simulink model "Simulator_Case_9"  (R2024a)
settings: Solver=VariableStepAuto  StartTime=0.0  StopTime=1400  RelTol=1e-3
values from neighbouring files (symbols this model uses):
  Declination_Sigean = 2.116*(pi/180)    (= 0.0369311669722)    [Parametrization_Simulation_Case_9.m]
  Position_Initial_X = Waypoints_X(1)    [Parametrization_Simulation_Case_9.m]
  Position_Initial_Y = Waypoints_Y(1)    [Parametrization_Simulation_Case_9.m]
  Time_Period_Sampling = 0.1    [Parametrization_Simulation_Case_9.m]
  Velocity_Norm_Ship_Initial = 6/3.6    (= 1.66666666667)    [Parametrization_Simulation_Case_9.m]
undefined symbols (not defined in the file or in its folder): Damping_Coefficient, Damping_Factor_Waves, Density_Water_Salted, Draft_Depth, Drag_Coefficient, Gain_Filter, Inertia_Moment, Length_Ship, Longeron_Area, Mass_Ship, Pulsation_Natural, Pulsation_Wave, Rudder_Angle_Maximal, Rudder_Angle_Minimal, Rudder_Rate_Maximal, Rudder_Rate_Minimal, Static_Gain_Nomoto, Time_Constant_Total, Waypoints
libraries: cstblocks x2, simulink_extras x1
(part 1 of 2)
settings Model: Creator=gerar  LastModifiedBy=gerar
settings DebuggingCC: UnderSpecifiedDimensionMsg=warning

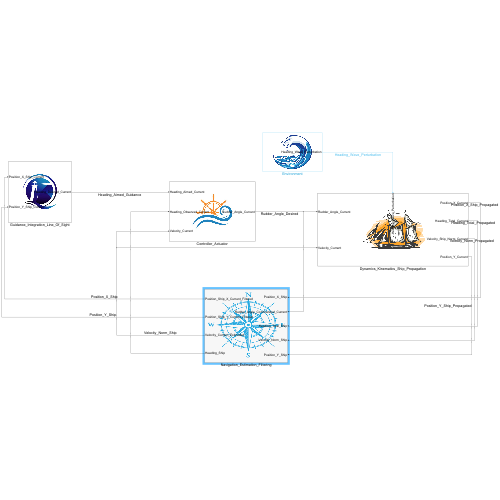
[thumbnail: Simulink's stored preview of the top-level diagram]
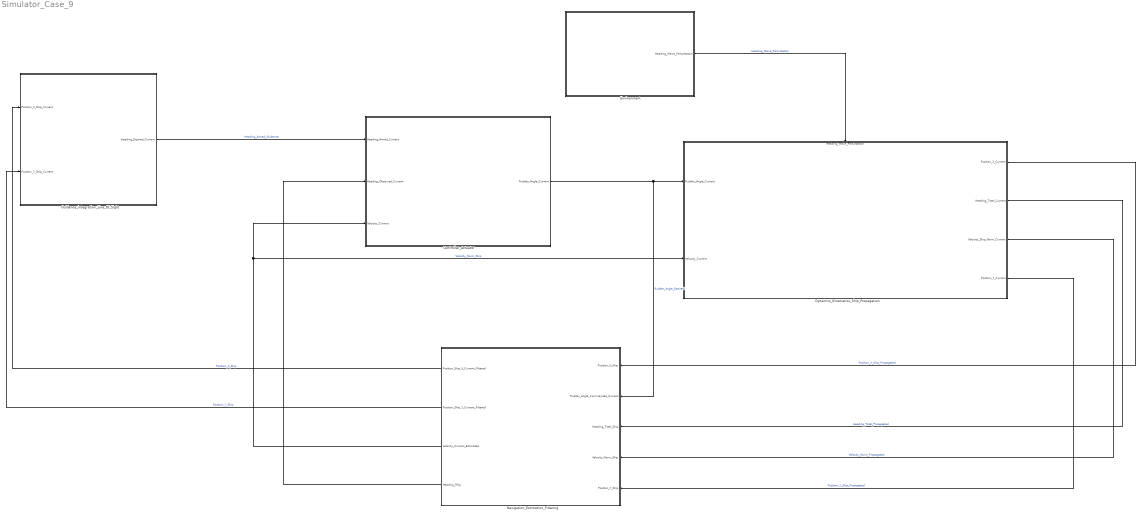
== system Simulator_Case_9 ==
  Controller_Actuator : Subsystem
      mask Display: image('Rudder3.jpg');
  Dynamics_Kinematics_Ship_Propagation : Subsystem
      settings: PortSchema="{\"entries\":[{\"content\":{\"sides\":[{\"content\":{\"connectorIds\":[\"In1\",\"In2\"]},\"type\":\"ConnectorPlacement.EquallySpacedRectSide\",\"uuid\":\"15ab685c-7974-4319-9f6c-957ada7f76c2\"},{\"content\":{\"connectorIds\":[\"Out1\",\"Out2\",\"Out3\",\"Out4\"],\"side\":\"RIGHT\"},\"type\":\"ConnectorPlacement.EquallySpacedRectSide\",\"uuid\":\"012aae79-88c5-42c2-86b9-e231f4da87b9\"},{\"content\":{\"connectorIds\":[\"In3\"],\"side\":\"TOP\"},\"type\":\"ConnectorPlacement.EquallySpacedRectSide\",\"uuid\":\"7672cff3-9f29-4819-a889-c5ff0e6add92\"}]},\"type\":\"ConnectorPlacement.EquallySpacedConnector\",\"uuid\":\"ccb47c3f-4c98-48cb-bcca-80a3d04d13a2\"}],\"packageUris\":[\"http://schema.mathworks.com/mf0/Connector/R2020b\"],\"version\":\"1.0\"}"
      mask Display: image('ship2.png');
  Environment : Subsystem
      mask Display: image('Wave2.png');
  Guidance_Integration_Line_Of_Sight : Subsystem
      mask Display: image('phare4.jpg');
  Navigation_Estimation_Filtering : Subsystem
      mask Display: image('compass4.png');
  wires:
  Navigation_Estimation_Filtering/1(Position_Ship_X_Current_Filtered) -> Guidance_Integration_Line_Of_Sight/1(Position_X_Ship_Current)  "Position_X_Ship"
  Navigation_Estimation_Filtering/2(Position_Ship_Y_Current_Filtered) -> Guidance_Integration_Line_Of_Sight/2(Position_Y_Ship_Current)  "Position_Y_Ship"
  Guidance_Integration_Line_Of_Sight/1(Heading_Desired_Current) -> Controller_Actuator/1(Heading_Aimed_Current)  "Heading_Aimed_Guidance"
  Navigation_Estimation_Filtering/3(Velocity_Current_Estimated) -> Dynamics_Kinematics_Ship_Propagation/2(Velocity_Current), Controller_Actuator/3(Velocity_Current)  "Velocity_Norm_Ship"
  Controller_Actuator/1(Rudder_Angle_Current) -> Navigation_Estimation_Filtering/2(Rudder_Angle_Commanded_Current), Dynamics_Kinematics_Ship_Propagation/1(Rudder_Angle_Current)  "Rudder_Angle_Desired"
  Environment/1(Heading_Wave_Perturbation) -> Dynamics_Kinematics_Ship_Propagation/3(Heading_Wave_Perturbation)  "Heading_Wave_Perturbation"
  Dynamics_Kinematics_Ship_Propagation/1(Position_X_Current) -> Navigation_Estimation_Filtering/1(Position_X_Ship)  "Position_X_Ship_Propagated"
  Dynamics_Kinematics_Ship_Propagation/2(Heading_Total_Current) -> Navigation_Estimation_Filtering/3(Heading_Total_Ship)  "Heading_Total_Propagated"
  Dynamics_Kinematics_Ship_Propagation/3(Velocity_Ship_Norm_Current) -> Navigation_Estimation_Filtering/4(Velocity_Norm_Ship)  "Velocity_Norm_Propagated"
  Dynamics_Kinematics_Ship_Propagation/4(Position_Y_Current) -> Navigation_Estimation_Filtering/5(Position_Y_Ship)  "Position_Y_Ship_Propagated"
  Navigation_Estimation_Filtering/4(Heading_Ship) -> Controller_Actuator/2(Heading_Observed_Current)

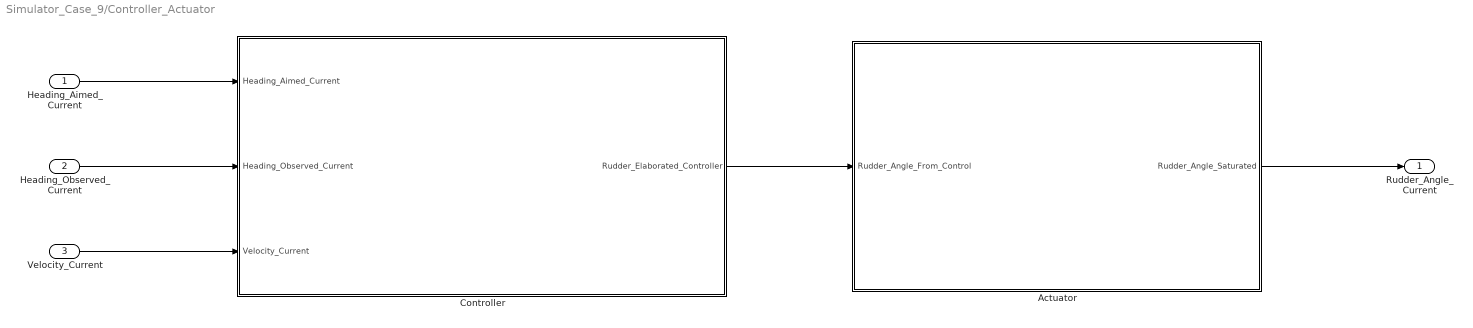
== system Simulator_Case_9/Controller_Actuator ==
  Heading_Aimed_Current : Inport
  Heading_Observed_Current : Inport  Port=2
  Velocity_Current : Inport  Port=3
  Actuator : Subsystem
  Controller : Subsystem
  Rudder_Angle_Current : Outport
  wires:
  Heading_Aimed_Current/1 -> Controller/1(Heading_Aimed_Current)
  Heading_Observed_Current/1 -> Controller/2(Heading_Observed_Current)
  Velocity_Current/1 -> Controller/3(Velocity_Current)
  Controller/1(Rudder_Elaborated_Controller) -> Actuator/1(Rudder_Angle_From_Control)
  Actuator/1(Rudder_Angle_Saturated) -> Rudder_Angle_Current/1

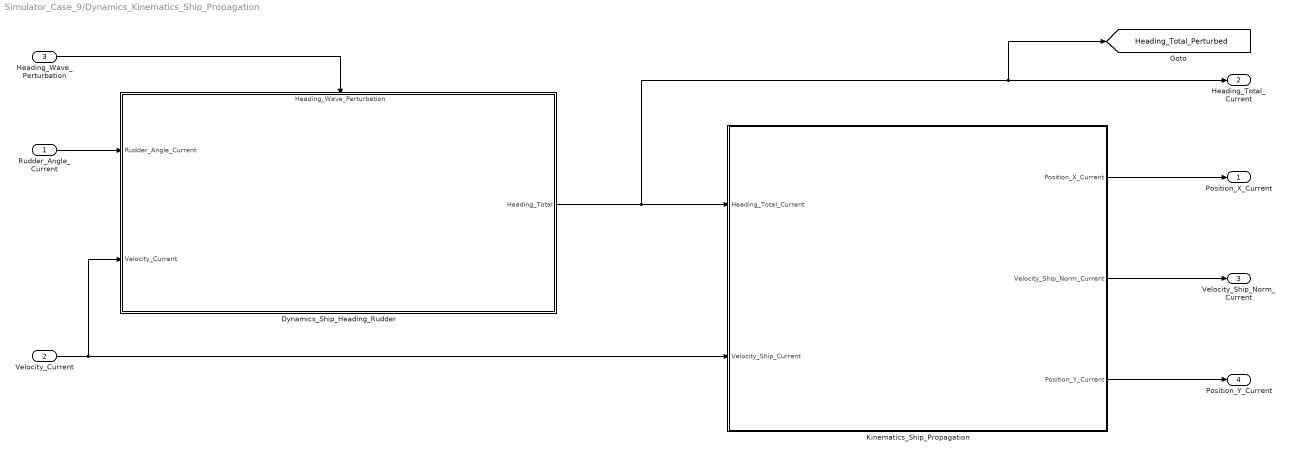
== system Simulator_Case_9/Dynamics_Kinematics_Ship_Propagation ==
  Rudder_Angle_Current : Inport
  Velocity_Current : Inport  Port=2
  Heading_Wave_Perturbation : Inport  Port=3
  Dynamics_Ship_Heading_Rudder : Subsystem
      settings: PortSchema="{\"entries\":[{\"content\":{\"sides\":[{\"content\":{\"connectorIds\":[\"In1\",\"In2\"]},\"type\":\"ConnectorPlacement.EquallySpacedRectSide\",\"uuid\":\"5eab7870-9471-4536-8507-22041873c494\"},{\"content\":{\"connectorIds\":[\"Out1\"],\"side\":\"RIGHT\"},\"type\":\"ConnectorPlacement.EquallySpacedRectSide\",\"uuid\":\"f266833a-c986-4c85-b5bf-5f6330a2f0dc\"},{\"content\":{\"connectorIds\":[\"In3\"],\"side\":\"TOP\"},\"type\":\"ConnectorPlacement.EquallySpacedRectSide\",\"uuid\":\"9dc2f366-9cc9-4ae6-8111-85e400a47094\"}]},\"type\":\"ConnectorPlacement.EquallySpacedConnector\",\"uuid\":\"570359d0-6206-4da5-90c2-7e8bebb6ea91\"}],\"packageUris\":[\"http://schema.mathworks.com/mf0/Connector/R2020b\"],\"version\":\"1.0\"}"
  Kinematics_Ship_Propagation : Subsystem
  Position_X_Current : Outport
  Heading_Total_Current : Outport  Port=2
  Velocity_Ship_Norm_Current : Outport  Port=3
  Position_Y_Current : Outport  Port=4
  tag scope: Heading_Total_Perturbed=global
  wires:
  Dynamics_Ship_Heading_Rudder/1(Heading_Total) -> [Heading_Total_Perturbed], Heading_Total_Current/1, Kinematics_Ship_Propagation/1(Heading_Total_Current)
  Kinematics_Ship_Propagation/1(Position_X_Current) -> Position_X_Current/1
  Velocity_Current/1 -> Kinematics_Ship_Propagation/2(Velocity_Ship_Current), Dynamics_Ship_Heading_Rudder/2(Velocity_Current)
  Rudder_Angle_Current/1 -> Dynamics_Ship_Heading_Rudder/1(Rudder_Angle_Current)
  Heading_Wave_Perturbation/1 -> Dynamics_Ship_Heading_Rudder/3(Heading_Wave_Perturbation)
  Kinematics_Ship_Propagation/3(Position_Y_Current) -> Position_Y_Current/1
  Kinematics_Ship_Propagation/2(Velocity_Ship_Norm_Current) -> Velocity_Ship_Norm_Current/1

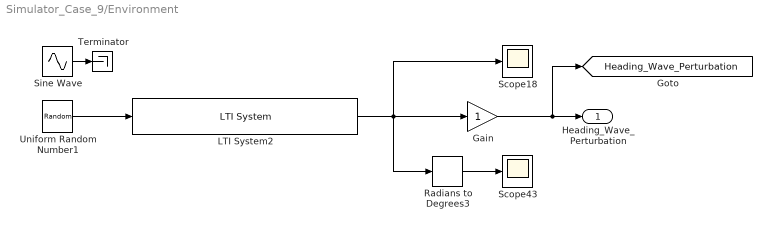
== system Simulator_Case_9/Environment ==
  Gain : Gain
  LTI System2 : cstblocks/LTI System  sys=Wave_Transfer_Function  IC=[]  PadeOrder=0
  Radians to Degrees3 : simulink_extras/Transformations/Radians to Degrees
  Scope18 : Scope
  Scope43 : Scope
  Sine Wave : Sin  Amplitude=6*(pi/180)  Frequency=1.2  SampleTime=0
  Terminator : Terminator
  Uniform Random Number1 : UniformRandomNumber  Minimum=-17*(pi/180)  Maximum=17*(pi/180)  SampleTime=Time_Period_Sampling
  Heading_Wave_Perturbation : Outport
  tag scope: Heading_Wave_Perturbation=global
  wires:
  LTI System2/1 -> Gain/1, Radians to Degrees3/1, Scope18/1
  Radians to Degrees3/1 -> Scope43/1
  Gain/1 -> [Heading_Wave_Perturbation], Heading_Wave_Perturbation/1
  Uniform Random Number1/1 -> LTI System2/1
  Sine Wave/1 -> Terminator/1

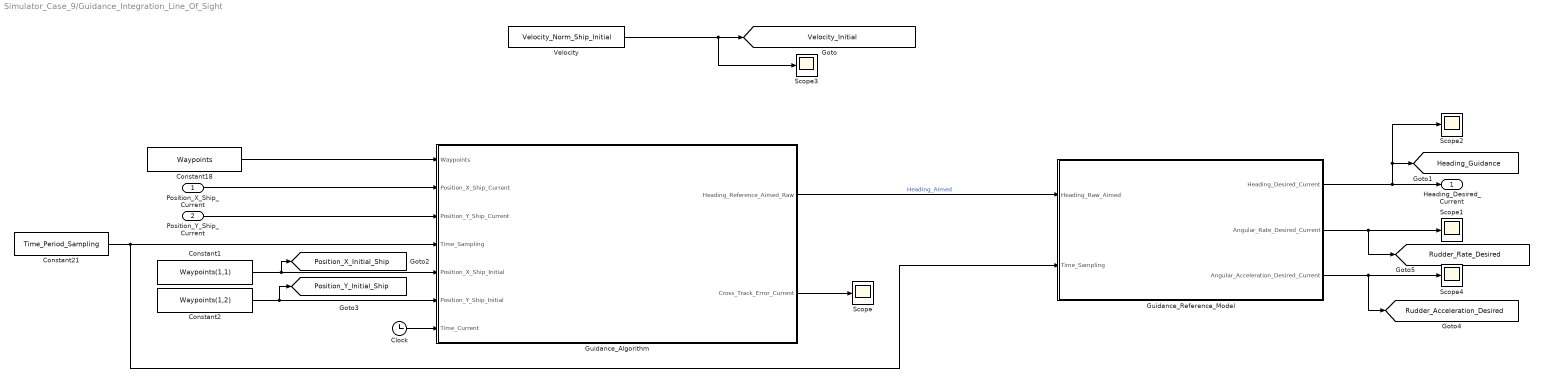
== system Simulator_Case_9/Guidance_Integration_Line_Of_Sight ==
  Position_X_Ship_Current : Inport
  Position_Y_Ship_Current : Inport  Port=2
  Clock : Clock
  Constant1 : Constant  Value=Waypoints(1,1)
  Constant18 : Constant  Value=Waypoints
  Constant2 : Constant  Value=Waypoints(1,2)
  Constant21 : Constant  Value=Time_Period_Sampling
  Guidance_Algorithm : MATLAB Function  TreatAsAtomicUnit=on  SystemSampleTime=Time_Period_Sampling
  Guidance_Reference_Model : MATLAB Function  TreatAsAtomicUnit=on  SystemSampleTime=Time_Period_Sampling
  Scope{,1..4} (5 alike) : Scope
  Velocity : Constant  Value=Velocity_Norm_Ship_Initial
  Heading_Desired_Current : Outport
  tag scope: Heading_Guidance=global, Position_X_Initial_Ship=global, Position_Y_Initial_Ship=global, Rudder_Acceleration_Desired=global, Rudder_Rate_Desired=global, Velocity_Initial=global
  wires:
  Guidance_Algorithm/2(Cross_Track_Error_Current) -> Scope/1
  Constant21/1 -> Guidance_Algorithm/4(Time_Sampling), Guidance_Reference_Model/2(Time_Sampling)
  Guidance_Reference_Model/2(Angular_Rate_Desired_Current) -> [Rudder_Rate_Desired], Scope1/1
  Constant18/1 -> Guidance_Algorithm/1(Waypoints)
  Guidance_Algorithm/1(Heading_Reference_Aimed_Raw) -> Guidance_Reference_Model/1(Heading_Raw_Aimed)  "Heading_Aimed"
  Guidance_Reference_Model/1(Heading_Desired_Current) -> Heading_Desired_Current/1, Scope2/1, [Heading_Guidance]
  Position_Y_Ship_Current/1 -> Guidance_Algorithm/3(Position_Y_Ship_Current)
  Position_X_Ship_Current/1 -> Guidance_Algorithm/2(Position_X_Ship_Current)
  Constant1/1 -> [Position_X_Initial_Ship], Guidance_Algorithm/5(Position_X_Ship_Initial)
  Constant2/1 -> [Position_Y_Initial_Ship], Guidance_Algorithm/6(Position_Y_Ship_Initial)
  Clock/1 -> Guidance_Algorithm/7(Time_Current)
  Velocity/1 -> Scope3/1, [Velocity_Initial]
  Guidance_Reference_Model/3(Angular_Acceleration_Desired_Current) -> [Rudder_Acceleration_Desired], Scope4/1

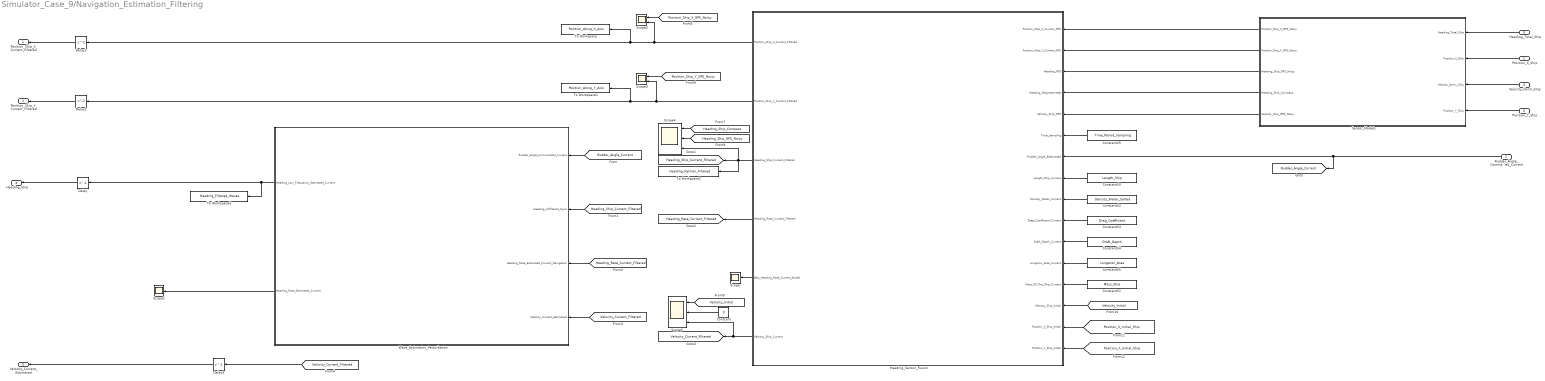
== system Simulator_Case_9/Navigation_Estimation_Filtering ==
  Position_X_Ship : Inport
  Rudder_Angle_Commanded_Current : Inport  Port=2
  Heading_Total_Ship : Inport  Port=3
  Velocity_Norm_Ship : Inport  Port=4
  Position_Y_Ship : Inport  Port=5
  Constant : Constant  Value=0
  Constant25 : Constant  Value=Time_Period_Sampling
  Constant50 : Constant  Value=Length_Ship
  Constant51 : Constant  Value=Mass_Ship
  Constant52 : Constant  Value=Density_Water_Salted
  Constant53 : Constant  Value=Drag_Coefficient
  Constant54 : Constant  Value=Draft_Depth
  Constant55 : Constant  Value=Longeron_Area
  Delay{,1..3} (4 alike) : Delay  DelayLength=1  InputProcessing=Columns as channels (frame based)  SampleTime=Time_Period_Sampling
  Heading_Sensor_Fusion : MATLAB Function  TreatAsAtomicUnit=on  SystemSampleTime=Time_Period_Sampling
  Scope : Scope
  Scope1 : Scope
  Scope2 : Scope  NumInputPorts=2
  Scope3 : Scope  NumInputPorts=2
  Scope4 : Scope  NumInputPorts=3
  Scope5 : Scope  NumInputPorts=3
  Sensor_Models : Subsystem
  To Workspace : ToWorkspace  VariableName=Position_Along_X_Axis  SaveFormat=Timeseries  SampleTime=-1
  To Workspace1 : ToWorkspace  VariableName=Position_Along_Y_Axis  SaveFormat=Timeseries  SampleTime=-1
  To Workspace2 : ToWorkspace  VariableName=Heading_Kalman_Filtered  SaveFormat=Timeseries  SampleTime=-1
  To Workspace3 : ToWorkspace  VariableName=Heading_Filtered_Waves  SaveFormat=Timeseries  SampleTime=-1
  Wave_Estimation_Perturbation : Subsystem
  Position_Ship_X_Current_Filtered : Outport
  Position_Ship_Y_Current_Filtered : Outport  Port=2
  Velocity_Current_Estimated : Outport  Port=3
  Heading_Ship : Outport  Port=4
  tag scope: Heading_Rate_Current_Filtered=global, Heading_Ship_Current_Filtered=global, Rudder_Angle_Current=global, Velocity_Current_Filtered=global
  wires:
  Heading_Sensor_Fusion/5(Bias_Heading_Rate_Current_Model) -> Scope/1
  Heading_Total_Ship/1 -> Sensor_Models/1(Heading_Total_Ship)
  Constant25/1 -> Heading_Sensor_Fusion/6(Time_Sampling)
  Constant55/1 -> Heading_Sensor_Fusion/12(Longeron_Area_Current)
  Sensor_Models/4(Heading_Ship_Compass) -> Heading_Sensor_Fusion/4(Heading_Magnetometer)
  Constant51/1 -> Heading_Sensor_Fusion/13(Mass_Of_The_Ship_Current)
  Sensor_Models/1(Position_Ship_X_GPS_Noisy) -> Heading_Sensor_Fusion/1(Position_Ship_X_Current_GPS)
  Sensor_Models/2(Position_Ship_Y_GPS_Noisy) -> Heading_Sensor_Fusion/2(Position_Ship_Y_Current_GPS)
  Velocity_Norm_Ship/1 -> Sensor_Models/3(Velocity_Norm_Ship)
  Sensor_Models/3(Heading_Ship_GPS_Noisy) -> Heading_Sensor_Fusion/3(Heading_GPS)
  Sensor_Models/5(Velocity_Ship_GPS_Noisy) -> Heading_Sensor_Fusion/5(Velocity_Ship_GPS)
  Constant54/1 -> Heading_Sensor_Fusion/11(Draft_Depth_Current)
  Constant50/1 -> Heading_Sensor_Fusion/8(Length_Ship_Current)
  Position_X_Ship/1 -> Sensor_Models/2(Position_X_Ship)
  Constant52/1 -> Heading_Sensor_Fusion/9(Density_Water_Current)
  Constant53/1 -> Heading_Sensor_Fusion/10(Drag_Coefficient_Current)
  Wave_Estimation_Perturbation/2(Heading_Rate_Estimated_Current) -> Scope1/1
  Wave_Estimation_Perturbation/1(Heading_Low_Frequency_Estimated_Current) -> To Workspace3/1, Delay/1
  Heading_Sensor_Fusion/2(Position_Ship_Y_Current_Filtered) -> Scope3/2, To Workspace1/1, Delay2/1
  Heading_Sensor_Fusion/1(Position_Ship_X_Current_Filtered) -> Scope2/2, To Workspace/1, Delay1/1
  Rudder_Angle_Commanded_Current/1 -> [Rudder_Angle_Current], Heading_Sensor_Fusion/7(Rudder_Angle_Elaborated)
  Position_Y_Ship/1 -> Sensor_Models/4(Position_Y_Ship)
  [Rudder_Angle_Current] -> Wave_Estimation_Perturbation/1(Rudder_Angle_Commanded_Current)
  Heading_Sensor_Fusion/3(Heading_Ship_Current_Filtered) -> To Workspace2/1, Scope4/3, [Heading_Ship_Current_Filtered]
  [Heading_Ship_Current_Filtered] -> Wave_Estimation_Perturbation/2(Heading_Unfiltered_Input)
  Heading_Sensor_Fusion/4(Heading_Rate_Current_Filtered) -> [Heading_Rate_Current_Filtered]
  [Heading_Rate_Current_Filtered] -> Wave_Estimation_Perturbation/3(Heading_Rate_Estimated_Current_Navigation)
  Heading_Sensor_Fusion/6(Velocity_Ship_Current) -> Scope5/3, [Velocity_Current_Filtered]
  [Velocity_Current_Filtered] -> Wave_Estimation_Perturbation/4(Velocity_Current_Estimated)
  [Velocity_Current_Filtered] -> Delay3/1
  [Position_Ship_X_GPS_Noisy] -> Scope2/1
  [Position_Ship_Y_GPS_Noisy] -> Scope3/1
  [Heading_Ship_Compass] -> Scope4/1
  [Heading_Ship_GPS_Noisy] -> Scope4/2
  [Velocity_Initial] -> Scope5/1
  Constant/1 -> Scope5/2
  [Velocity_Initial] -> Heading_Sensor_Fusion/14(Velocity_Ship_Initial)
  [Position_X_Initial_Ship] -> Heading_Sensor_Fusion/15(Position_X_Ship_Initial)
  [Position_Y_Initial_Ship] -> Heading_Sensor_Fusion/16(Position_Y_Ship_Initial)
  Delay1/1 -> Position_Ship_X_Current_Filtered/1
  Delay2/1 -> Position_Ship_Y_Current_Filtered/1
  Delay/1 -> Heading_Ship/1
  Delay3/1 -> Velocity_Current_Estimated/1

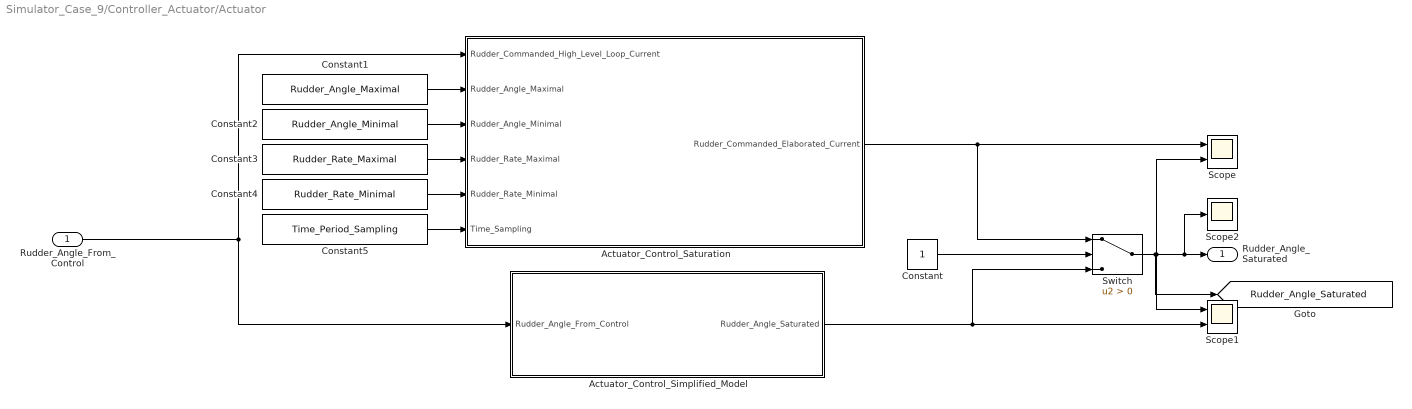
== system Simulator_Case_9/Controller_Actuator/Actuator ==
  Rudder_Angle_From_Control : Inport
  Actuator_Control_Saturation : MATLAB Function  TreatAsAtomicUnit=on  SystemSampleTime=Time_Period_Sampling
  Actuator_Control_Simplified_Model : Subsystem
  Constant : Constant
  Constant1 : Constant  Value=Rudder_Angle_Maximal
  Constant2 : Constant  Value=Rudder_Angle_Minimal
  Constant3 : Constant  Value=Rudder_Rate_Maximal
  Constant4 : Constant  Value=Rudder_Rate_Minimal
  Constant5 : Constant  Value=Time_Period_Sampling
  Scope : Scope  NumInputPorts=2
  Scope1 : Scope  NumInputPorts=2
  Scope2 : Scope
  Switch : Switch  Criteria=u2 > Threshold  SaturateOnIntegerOverflow=off  InputSameDT=off
  Rudder_Angle_Saturated : Outport
  tag scope: Rudder_Angle_Saturated=global
  wires:
  Constant/1 -> Switch/2
  Constant5/1 -> Actuator_Control_Saturation/6(Time_Sampling)
  Actuator_Control_Simplified_Model/1(Rudder_Angle_Saturated) -> Scope1/2, Switch/3
  Actuator_Control_Saturation/1(Rudder_Commanded_Elaborated_Current) -> Scope/1, Switch/1
  Constant4/1 -> Actuator_Control_Saturation/5(Rudder_Rate_Minimal)
  Rudder_Angle_From_Control/1 -> Actuator_Control_Simplified_Model/1(Rudder_Angle_From_Control), Actuator_Control_Saturation/1(Rudder_Commanded_High_Level_Loop_Current)
  Constant2/1 -> Actuator_Control_Saturation/3(Rudder_Angle_Minimal)
  Constant1/1 -> Actuator_Control_Saturation/2(Rudder_Angle_Maximal)
  Constant3/1 -> Actuator_Control_Saturation/4(Rudder_Rate_Maximal)
  Switch/1 -> Scope2/1, Rudder_Angle_Saturated/1, Scope1/1, Scope/2, [Rudder_Angle_Saturated]

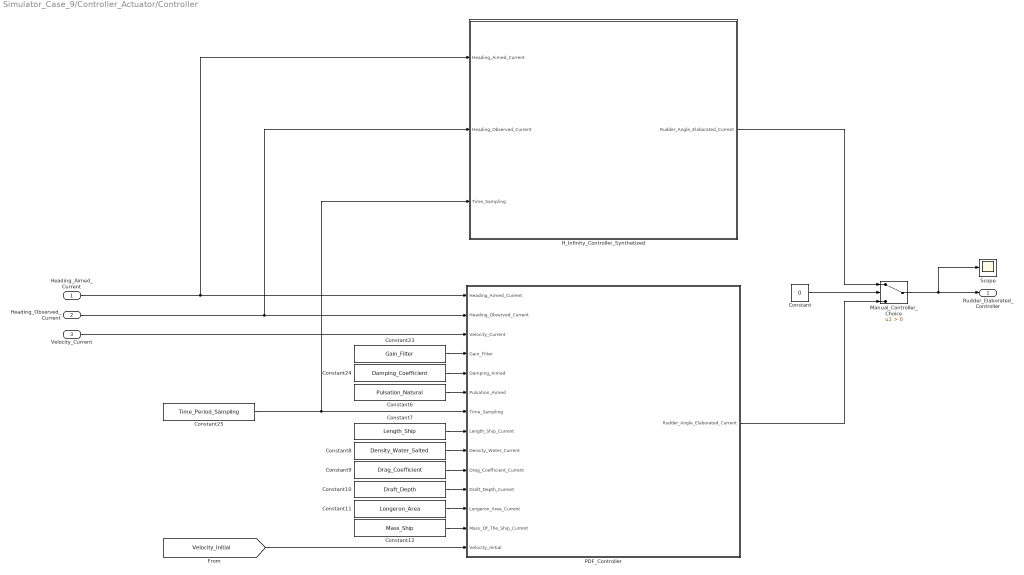
== system Simulator_Case_9/Controller_Actuator/Controller ==
  Heading_Aimed_Current : Inport
  Heading_Observed_Current : Inport  Port=2
  Velocity_Current : Inport  Port=3
  Constant : Constant  Value=0
  Constant10 : Constant  Value=Draft_Depth
  Constant11 : Constant  Value=Longeron_Area
  Constant12 : Constant  Value=Mass_Ship
  Constant23 : Constant  Value=Gain_Filter
  Constant24 : Constant  Value=Damping_Coefficient
  Constant25 : Constant  Value=Time_Period_Sampling
  Constant6 : Constant  Value=Pulsation_Natural
  Constant7 : Constant  Value=Length_Ship
  Constant8 : Constant  Value=Density_Water_Salted
  Constant9 : Constant  Value=Drag_Coefficient
  H_Infinity_Controller_Synthetized : MATLAB Function  TreatAsAtomicUnit=on  SystemSampleTime=Time_Period_Sampling
  Manual_Controller_Choice : Switch  Criteria=u2 > Threshold  SaturateOnIntegerOverflow=off  InputSameDT=off
  PDF_Controller : MATLAB Function  TreatAsAtomicUnit=on  SystemSampleTime=Time_Period_Sampling
  Scope : Scope
  Rudder_Elaborated_Controller : Outport
  wires:
  Constant24/1 -> PDF_Controller/5(Damping_Aimed)
  Constant9/1 -> PDF_Controller/10(Drag_Coefficient_Current)
  Velocity_Current/1 -> PDF_Controller/3(Velocity_Current)
  Constant6/1 -> PDF_Controller/6(Pulsation_Aimed)
  Constant12/1 -> PDF_Controller/13(Mass_Of_The_Ship_Current)
  Constant10/1 -> PDF_Controller/11(Draft_Depth_Current)
  Constant7/1 -> PDF_Controller/8(Length_Ship_Current)
  Constant25/1 -> H_Infinity_Controller_Synthetized/3(Time_Sampling), PDF_Controller/7(Time_Sampling)
  Constant23/1 -> PDF_Controller/4(Gain_Filter)
  [Velocity_Initial] -> PDF_Controller/14(Velocity_Initial)
  Constant8/1 -> PDF_Controller/9(Density_Water_Current)
  Constant11/1 -> PDF_Controller/12(Longeron_Area_Current)
  Heading_Observed_Current/1 -> PDF_Controller/2(Heading_Observed_Current), H_Infinity_Controller_Synthetized/2(Heading_Observed_Current)
  Constant/1 -> Manual_Controller_Choice/2
  Heading_Aimed_Current/1 -> PDF_Controller/1(Heading_Aimed_Current), H_Infinity_Controller_Synthetized/1(Heading_Aimed_Current)
  H_Infinity_Controller_Synthetized/1(Rudder_Angle_Elaborated_Current) -> Manual_Controller_Choice/1
  PDF_Controller/1(Rudder_Angle_Elaborated_Current) -> Manual_Controller_Choice/3
  Manual_Controller_Choice/1 -> Rudder_Elaborated_Controller/1, Scope/1

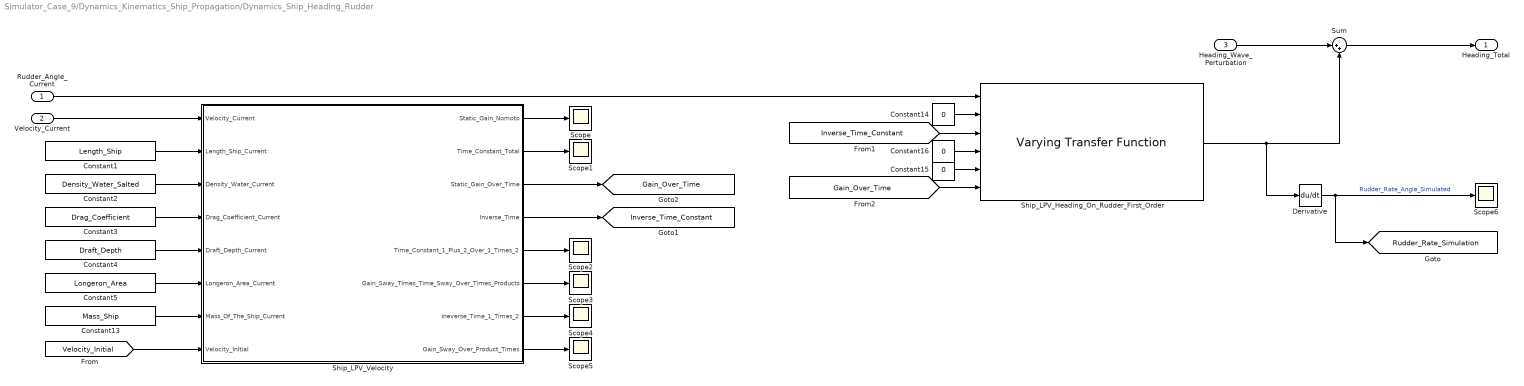
== system Simulator_Case_9/Dynamics_Kinematics_Ship_Propagation/Dynamics_Ship_Heading_Rudder ==
  Rudder_Angle_Current : Inport
  Velocity_Current : Inport  Port=2
  Heading_Wave_Perturbation : Inport  Port=3
  Constant1 : Constant  Value=Length_Ship
  Constant13 : Constant  Value=Mass_Ship
  Constant14 : Constant  Value=0
  Constant15 : Constant  Value=0
  Constant16 : Constant  Value=0
  Constant2 : Constant  Value=Density_Water_Salted
  Constant3 : Constant  Value=Drag_Coefficient
  Constant4 : Constant  Value=Draft_Depth
  Constant5 : Constant  Value=Longeron_Area
  Derivative : Derivative
  Scope{,1..6} (7 alike) : Scope
  Ship_LPV_Heading_On_Rudder_First_Order : cstblocks/Linear Parameter Varying/Varying Transfer Function  N=2  Feedthrough=on
  Ship_LPV_Velocity : MATLAB Function  TreatAsAtomicUnit=on
  Sum : Sum  Inputs=|++
  Heading_Total : Outport
  tag scope: Gain_Over_Time=global, Inverse_Time_Constant=global, Rudder_Rate_Simulation=global
  wires:
  Ship_LPV_Velocity/7(Ineverse_Time_1_Times_2) -> Scope4/1
  Ship_LPV_Heading_On_Rudder_First_Order/1 -> Sum/2, Derivative/1
  Constant15/1 -> Ship_LPV_Heading_On_Rudder_First_Order/5
  [Inverse_Time_Constant] -> Ship_LPV_Heading_On_Rudder_First_Order/3
  Constant2/1 -> Ship_LPV_Velocity/3(Density_Water_Current)
  [Gain_Over_Time] -> Ship_LPV_Heading_On_Rudder_First_Order/6
  Ship_LPV_Velocity/1(Static_Gain_Nomoto) -> Scope/1
  Constant5/1 -> Ship_LPV_Velocity/6(Longeron_Area_Current)
  [Velocity_Initial] -> Ship_LPV_Velocity/8(Velocity_Initial)
  Ship_LPV_Velocity/2(Time_Constant_Total) -> Scope1/1
  Ship_LPV_Velocity/8(Gain_Sway_Over_Product_Times) -> Scope5/1
  Constant14/1 -> Ship_LPV_Heading_On_Rudder_First_Order/2
  Constant16/1 -> Ship_LPV_Heading_On_Rudder_First_Order/4
  Ship_LPV_Velocity/4(Inverse_Time) -> [Inverse_Time_Constant]
  Ship_LPV_Velocity/6(Gain_Sway_Times_Time_Sway_Over_Times_Products) -> Scope3/1
  Ship_LPV_Velocity/3(Static_Gain_Over_Time) -> [Gain_Over_Time]
  Heading_Wave_Perturbation/1 -> Sum/1
  Constant1/1 -> Ship_LPV_Velocity/2(Length_Ship_Current)
  Constant13/1 -> Ship_LPV_Velocity/7(Mass_Of_The_Ship_Current)
  Constant3/1 -> Ship_LPV_Velocity/4(Drag_Coefficient_Current)
  Rudder_Angle_Current/1 -> Ship_LPV_Heading_On_Rudder_First_Order/1
  Constant4/1 -> Ship_LPV_Velocity/5(Draft_Depth_Current)
  Ship_LPV_Velocity/5(Time_Constant_1_Plus_2_Over_1_Times_2) -> Scope2/1
  Derivative/1 -> [Rudder_Rate_Simulation], Scope6/1  "Rudder_Rate_Angle_Simulated"
  Velocity_Current/1 -> Ship_LPV_Velocity/1(Velocity_Current)
  Sum/1 -> Heading_Total/1

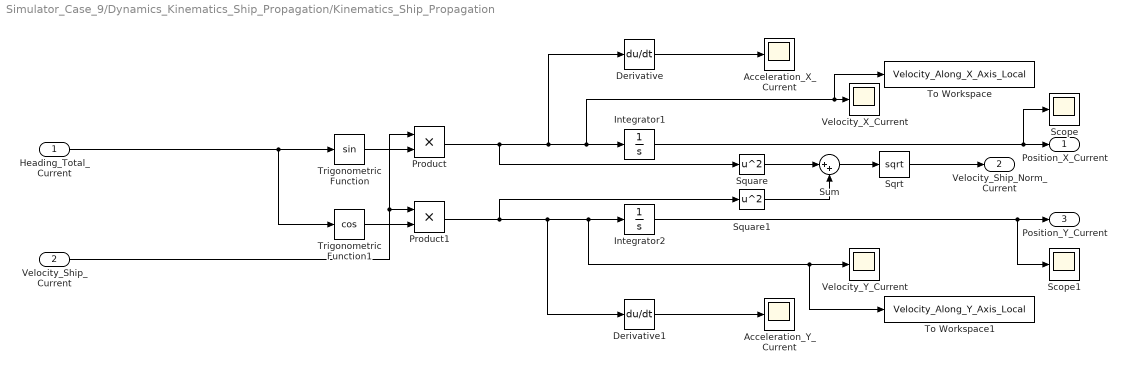
== system Simulator_Case_9/Dynamics_Kinematics_Ship_Propagation/Kinematics_Ship_Propagation ==
  Heading_Total_Current : Inport
  Velocity_Ship_Current : Inport  Port=2
  Acceleration_X_Current : Scope
  Acceleration_Y_Current : Scope
  Derivative : Derivative
  Derivative1 : Derivative
  Integrator1 : Integrator  InitialCondition=Position_Initial_X
  Integrator2 : Integrator  InitialCondition=Position_Initial_Y
  Product : Product
  Product1 : Product
  Scope : Scope
  Scope1 : Scope
  Sqrt : Sqrt
  Square : Math  Operator=square
  Square1 : Math  Operator=square
  Sum : Sum  Inputs=|++
  To Workspace : ToWorkspace  VariableName=Velocity_Along_X_Axis_Local  SaveFormat=Timeseries  SampleTime=-1
  To Workspace1 : ToWorkspace  VariableName=Velocity_Along_Y_Axis_Local  SaveFormat=Timeseries  SampleTime=-1
  Trigonometric Function : Trigonometry
  Trigonometric Function1 : Trigonometry  Operator=cos
  Velocity_X_Current : Scope
  Velocity_Y_Current : Scope
  Position_X_Current : Outport
  Velocity_Ship_Norm_Current : Outport  Port=2
  Position_Y_Current : Outport  Port=3
  wires:
  Product1/1 -> Square1/1, Derivative1/1, Velocity_Y_Current/1, To Workspace1/1, Integrator2/1
  Square/1 -> Sum/1
  Product/1 -> Square/1, Derivative/1, To Workspace/1, Velocity_X_Current/1, Integrator1/1
  Trigonometric Function/1 -> Product/2
  Heading_Total_Current/1 -> Trigonometric Function1/1, Trigonometric Function/1
  Velocity_Ship_Current/1 -> Product1/1, Product/1
  Square1/1 -> Sum/2
  Trigonometric Function1/1 -> Product1/2
  Sum/1 -> Sqrt/1
  Integrator1/1 -> Scope/1, Position_X_Current/1
  Integrator2/1 -> Scope1/1, Position_Y_Current/1
  Sqrt/1 -> Velocity_Ship_Norm_Current/1
  Derivative1/1 -> Acceleration_Y_Current/1
  Derivative/1 -> Acceleration_X_Current/1

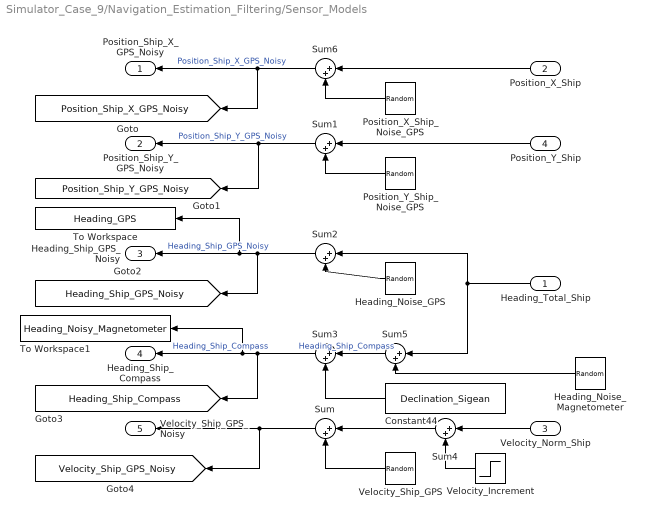
== system Simulator_Case_9/Navigation_Estimation_Filtering/Sensor_Models ==
  Heading_Total_Ship : Inport
  Position_X_Ship : Inport  Port=2
  Velocity_Norm_Ship : Inport  Port=3
  Position_Y_Ship : Inport  Port=4
  Constant44 : Constant  Value=Declination_Sigean
  Heading_Noise_GPS : UniformRandomNumber  Minimum=-5*(pi/180)  Maximum=5*(pi/180)  SampleTime=Time_Period_Sampling
  Heading_Noise_Magnetometer : UniformRandomNumber  Minimum=-2*(pi/180)  Maximum=2*(pi/180)  SampleTime=Time_Period_Sampling
  Position_X_Ship_Noise_GPS : UniformRandomNumber  Minimum=-2  Maximum=2  SampleTime=Time_Period_Sampling
  Position_Y_Ship_Noise_GPS : UniformRandomNumber  Minimum=-2  Maximum=2  SampleTime=Time_Period_Sampling
  Sum{,1..6} (7 alike) : Sum  Inputs=|++
  To Workspace : ToWorkspace  VariableName=Heading_GPS  SaveFormat=Timeseries  SampleTime=-1
  To Workspace1 : ToWorkspace  VariableName=Heading_Noisy_Magnetometer  SaveFormat=Timeseries  SampleTime=-1
  Velocity_Increment : Step  Time=300  After=0  SampleTime=0
  Velocity_Ship_GPS : UniformRandomNumber  Minimum=-0.1  Maximum=0.1  SampleTime=Time_Period_Sampling
  Position_Ship_X_GPS_Noisy : Outport
  Position_Ship_Y_GPS_Noisy : Outport  Port=2
  Heading_Ship_GPS_Noisy : Outport  Port=3
  Heading_Ship_Compass : Outport  Port=4
  Velocity_Ship_GPS_Noisy : Outport  Port=5
  tag scope: Heading_Ship_Compass=global, Heading_Ship_GPS_Noisy=global, Position_Ship_X_GPS_Noisy=global, Position_Ship_Y_GPS_Noisy=global, Velocity_Ship_GPS_Noisy=global
  wires:
  Position_X_Ship_Noise_GPS/1 -> Sum6/2
  Constant44/1 -> Sum3/2
  Position_Y_Ship/1 -> Sum1/1
  Velocity_Ship_GPS/1 -> Sum/2
  Position_Y_Ship_Noise_GPS/1 -> Sum1/2
  Sum/1 -> [Velocity_Ship_GPS_Noisy], Velocity_Ship_GPS_Noisy/1
  Heading_Noise_GPS/1 -> Sum2/2
  Sum1/1 -> [Position_Ship_Y_GPS_Noisy], Position_Ship_Y_GPS_Noisy/1  "Position_Ship_Y_GPS_Noisy"
  Sum2/1 -> [Heading_Ship_GPS_Noisy], Heading_Ship_GPS_Noisy/1, To Workspace/1  "Heading_Ship_GPS_Noisy"
  Sum6/1 -> [Position_Ship_X_GPS_Noisy], Position_Ship_X_GPS_Noisy/1  "Position_Ship_X_GPS_Noisy"
  Position_X_Ship/1 -> Sum6/1
  Sum3/1 -> [Heading_Ship_Compass], To Workspace1/1, Heading_Ship_Compass/1  "Heading_Ship_Compass"
  Sum4/1 -> Sum/1
  Velocity_Norm_Ship/1 -> Sum4/1
  Velocity_Increment/1 -> Sum4/2
  Heading_Total_Ship/1 -> Sum5/1, Sum2/1
  Sum5/1 -> Sum3/1  "Heading_Ship_Compass"
  Heading_Noise_Magnetometer/1 -> Sum5/2

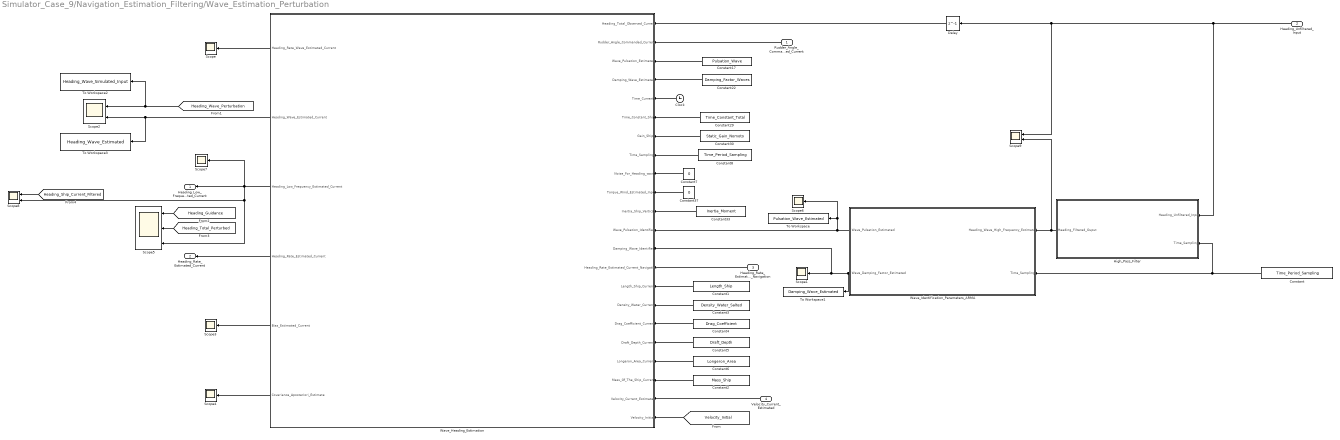
== system Simulator_Case_9/Navigation_Estimation_Filtering/Wave_Estimation_Perturbation ==
  Rudder_Angle_Commanded_Current : Inport
  Heading_Unfiltered_Input : Inport  Port=2
  Heading_Rate_Estimated_Current_Navigation : Inport  Port=3
  Velocity_Current_Estimated : Inport  Port=4
  Clock : Clock
  Constant : Constant  Value=Time_Period_Sampling
  Constant1 : Constant  Value=Length_Ship
  Constant17 : Constant  Value=Pulsation_Wave  SampleTime=Time_Period_Sampling
  Constant2 : Constant  Value=Mass_Ship
  Constant22 : Constant  Value=Damping_Factor_Waves  SampleTime=Time_Period_Sampling
  Constant29 : Constant  Value=Time_Constant_Total  SampleTime=Time_Period_Sampling
  Constant3 : Constant  Value=Density_Water_Salted
  Constant30 : Constant  Value=Static_Gain_Nomoto  SampleTime=Time_Period_Sampling
  Constant33 : Constant  Value=Inertia_Moment
  Constant37 : Constant  Value=0
  Constant4 : Constant  Value=Drag_Coefficient
  Constant5 : Constant  Value=Draft_Depth
  Constant6 : Constant  Value=Longeron_Area
  Constant7 : Constant  Value=0
  Constant8 : Constant  Value=Time_Period_Sampling
  Delay : Delay  DelayLength=1  InputProcessing=Columns as channels (frame based)  SampleTime=Time_Period_Sampling
  High_Pass_Filter : MATLAB Function  TreatAsAtomicUnit=on  SystemSampleTime=Time_Period_Sampling
  Scope{,1,3..4,6..7} (6 alike) : Scope
  Scope2 : Scope  NumInputPorts=2
  Scope5 : Scope  NumInputPorts=3
  Scope8 : Scope  NumInputPorts=2
  Scope9 : Scope  NumInputPorts=2
  To Workspace : ToWorkspace  VariableName=Pulsation_Wave_Estimated  SaveFormat=Timeseries  SampleTime=-1
  To Workspace1 : ToWorkspace  VariableName=Damping_Wave_Estimated  SaveFormat=Timeseries  SampleTime=-1
  To Workspace2 : ToWorkspace  VariableName=Heading_Wave_Simulated_Input  SaveFormat=Timeseries  SampleTime=-1
  To Workspace3 : ToWorkspace  VariableName=Heading_Wave_Estimated  SaveFormat=Timeseries  SampleTime=-1
  Wave_Heading_Estimation : MATLAB Function  TreatAsAtomicUnit=on  SystemSampleTime=Time_Period_Sampling
  Wave_Identification_Parameters_ARMA : MATLAB Function  TreatAsAtomicUnit=on  SystemSampleTime=Time_Period_Sampling
  Heading_Low_Frequency_Estimated_Current : Outport
  Heading_Rate_Estimated_Current : Outport  Port=2
  wires:
  Wave_Identification_Parameters_ARMA/2(Wave_Damping_Factor_Estimated) -> Wave_Heading_Estimation/13(Damping_Wave_Identified), Scope1/1, To Workspace1/1
  Constant7/1 -> Wave_Heading_Estimation/9(Noise_For_Heading_wave)
  Constant30/1 -> Wave_Heading_Estimation/7(Gain_Ship)
  Heading_Unfiltered_Input/1 -> High_Pass_Filter/1(Heading_Unfiltered_Input), Scope9/1, Delay/1
  Constant29/1 -> Wave_Heading_Estimation/6(Time_Constant_Ship)
  Wave_Identification_Parameters_ARMA/1(Wave_Pulsation_Estimated) -> Scope6/1, To Workspace/1, Wave_Heading_Estimation/12(Wave_Pulsation_Identified)
  Wave_Heading_Estimation/3(Heading_Low_Frequency_Estimated_Current) -> Scope7/1, Scope8/2, Scope5/3, Heading_Low_Frequency_Estimated_Current/1
  Constant4/1 -> Wave_Heading_Estimation/17(Drag_Coefficient_Current)
  Constant22/1 -> Wave_Heading_Estimation/4(Damping_Wave_Estimated)
  Rudder_Angle_Commanded_Current/1 -> Wave_Heading_Estimation/2(Rudder_Angle_Commanded_Current)
  Constant/1 -> Wave_Identification_Parameters_ARMA/2(Time_Sampling), High_Pass_Filter/2(Time_Sampling)
  Constant6/1 -> Wave_Heading_Estimation/19(Longeron_Area_Current)
  Constant33/1 -> Wave_Heading_Estimation/11(Inertia_Ship_Vertical)
  Constant3/1 -> Wave_Heading_Estimation/16(Density_Water_Current)
  [Velocity_Initial] -> Wave_Heading_Estimation/22(Velocity_Initial)
  Wave_Heading_Estimation/2(Heading_Wave_Estimated_Current) -> To Workspace3/1, Scope2/2
  Constant17/1 -> Wave_Heading_Estimation/3(Wave_Pulsation_Estimated)
  Constant8/1 -> Wave_Heading_Estimation/8(Time_Sampling)
  High_Pass_Filter/1(Heading_Filtered_Ouput) -> Scope9/2, Wave_Identification_Parameters_ARMA/1(Heading_Wave_High_Frequency_Estimated)
  Constant5/1 -> Wave_Heading_Estimation/18(Draft_Depth_Current)
  Wave_Heading_Estimation/4(Heading_Rate_Estimated_Current) -> Heading_Rate_Estimated_Current/1
  Constant37/1 -> Wave_Heading_Estimation/10(Torque_Wind_Estimated_Input)
  Delay/1 -> Wave_Heading_Estimation/1(Heading_Total_Observed_Current)
  Clock/1 -> Wave_Heading_Estimation/5(Time_Current)
  Constant2/1 -> Wave_Heading_Estimation/20(Mass_Of_The_Ship_Current)
  Constant1/1 -> Wave_Heading_Estimation/15(Length_Ship_Current)
  Wave_Heading_Estimation/1(Heading_Rate_Wave_Estimated_Current) -> Scope/1
  Wave_Heading_Estimation/5(Bias_Estimated_Current) -> Scope3/1
  Wave_Heading_Estimation/6(Covariance_Aposteriori_Estimate) -> Scope4/1
  Velocity_Current_Estimated/1 -> Wave_Heading_Estimation/21(Velocity_Current_Estimated)
  Heading_Rate_Estimated_Current_Navigation/1 -> Wave_Heading_Estimation/14(Heading_Rate_Estimated_Current_Navigation)
  [Heading_Wave_Perturbation] -> To Workspace2/1, Scope2/1
  [Heading_Guidance] -> Scope5/1
  [Heading_Total_Perturbed] -> Scope5/2
  [Heading_Ship_Current_Filtered] -> Scope8/1

== system Simulator_Case_9/Controller_Actuator/Actuator/Actuator_Control_Simplified_Model ==
  Rudder_Angle_From_Control : Inport
  Angular_Rate_Saturation : Saturate  UpperLimit=11*(pi/180)  LowerLimit=-11*(pi/180)
  Integrator : Integrator
  Rudder_Angle_Saturation : Saturate  UpperLimit=Rudder_Angle_Maximal  LowerLimit=-Rudder_Angle_Maximal
  Sum1 : Sum  Inputs=|+-
  Rudder_Angle_Saturated : Outport
  wires:
  Integrator/1 -> Rudder_Angle_Saturated/1, Sum1/2
  Rudder_Angle_From_Control/1 -> Rudder_Angle_Saturation/1
  Rudder_Angle_Saturation/1 -> Sum1/1
  Sum1/1 -> Angular_Rate_Saturation/1
  Angular_Rate_Saturation/1 -> Integrator/1

== matlab function Simulator_Case_9/Controller_Actuator/Actuator/Actuator_Control_Saturation ==
  data: Rudder_Commanded_High_Level_Loop_Current input; Rudder_Commanded_Elaborated_Current output; Rudder_Angle_Maximal input; Rudder_Angle_Minimal input; Rudder_Rate_Maximal input; Rudder_Rate_Minimal input; Time_Sampling input
function Rudder_Commanded_Elaborated_Current = Linear_Actuator_First_Order(Rudder_Commanded_High_Level_Loop_Current,...
                                                                           Rudder_Angle_Maximal,...
                                                                           Rudder_Angle_Minimal,...
                                                                           Rudder_Rate_Maximal,...
                                                                           Rudder_Rate_Minimal,...
                                                                           Time_Sampling)

% This function acts as a simplified model of a first Actuator version. It
% consists in a first saturation of the commanded rudder angle in terms of
% maximal and minimal angles value. And a second saturation in terms of maximal and
% minimal rudder angle rate.
Rudder_Commanded_Elaborated_Current = Rudder_Angle_Rate_Saturations(Rudder_Commanded_High_Level_Loop_Current,...
                                                                    Rudder_Angle_Maximal,...
                                                                    Rudder_Angle_Minimal,...
                                                                    Rudder_Rate_Maximal,...
                                                                    Rudder_Rate_Minimal,...
                                                                    Time_Sampling);

end

== matlab function Simulator_Case_9/Navigation_Estimation_Filtering/Wave_Estimation_Perturbation/Wave_Heading_Estimation ==
  data: Heading_Total_Observed_Current input; Rudder_Angle_Commanded_Current input; Wave_Pulsation_Estimated input; Damping_Wave_Estimated input; Time_Current input; Time_Constant_Ship input; Gain_Ship input; Time_Sampling input; Noise_For_Heading_wave input; Heading_Rate_Wave_Estimated_Current output; Heading_Wave_Estimated_Current output; Heading_Low_Frequency_Estimated_Current output; Heading_Rate_Estimated_Current output; Bias_Estimated_Current output; Covariance_Aposteriori_Estimate output; Torque_Wind_Estimated_Input input; Inertia_Ship_Vertical input; Wave_Pulsation_Identified input; Damping_Wave_Identified input; Heading_Rate_Estimated_Current_Navigation input; Length_Ship_Current input; Density_Water_Current input; Drag_Coefficient_Current input; Draft_Depth_Current input; Longeron_Area_Current input; Mass_Of_The_Ship_Current input; Velocity_Current_Estimated input; Velocity_Initial input
function [Heading_Rate_Wave_Estimated_Current,...
          Heading_Wave_Estimated_Current,...
          Heading_Low_Frequency_Estimated_Current,...
          Heading_Rate_Estimated_Current,...
          Bias_Estimated_Current,...
          Covariance_Aposteriori_Estimate]= Kalman_Filter_Wave_Estimation(Heading_Total_Observed_Current,...
                                                                          Rudder_Angle_Commanded_Current,...
                                                                          Wave_Pulsation_Estimated,...
                                                                          Damping_Wave_Estimated,...
                                                                          Time_Current,...
                                                                          Time_Constant_Ship,...
                                                                          Gain_Ship,...
                                                                          Time_Sampling,...
                                                                          Noise_For_Heading_wave,...
                                                                          Torque_Wind_Estimated_Input,...
                                                                          Inertia_Ship_Vertical,...
                                                                          Wave_Pulsation_Identified,...
                                                                          Damping_Wave_Identified,...
                                                                          Heading_Rate_Estimated_Current_Navigation,...
                                                                          Length_Ship_Current,...
                                                                          Density_Water_Current,...
                                                                          Drag_Coefficient_Current,...
                                                                          Draft_Depth_Current,...
                                                                          Longeron_Area_Current,...
                                                                          Mass_Of_The_Ship_Current,...
                                                                          Velocity_Current_Estimated,...
                                                                          Velocity_Initial)

% Time constant and ship static gain evolution in function of the velocity
% to be computed:
if Velocity_Current_Estimated == 0
    Velocity_Current_Estimated = Velocity_Initial;
end
Is_Estimation_Ship_Parameters = 1;
if Is_Estimation_Ship_Parameters
    [Static_Gain,Time_Constant] = Static_Gain_Time_Constant_Varying_Velocity_Embedded(Velocity_Current_Estimated,... % Considered to be the cleanest.
                                                                                      Length_Ship_Current,...
                                                                                      Density_Water_Current,...
                                                                                      Drag_Coefficient_Current,...
                                                                                      Draft_Depth_Current,...
                                                                                      Longeron_Area_Current,...
                                                                                      Mass_Of_The_Ship_Current);
else
    Static_Gain = Gain_Ship;
    Time_Constant = Time_Constant_Ship;
end

% Online Wave Observer Kalman algorithm for better wave high frequency
% filtering:
Is_Discretization_Euler = 1;
if Is_Discretization_Euler
    [Heading_Rate_Wave_Estimated_Current,...
     Heading_Wave_Estimated_Current,...
     Heading_Low_Frequency_Estimated_Current,...
     Heading_Rate_Estimated_Current,...
     Bias_Estimated_Current,...
     Covariance_Aposteriori_Estimate] = Kalman_Observer_Wave_Estimation_Dynamics(Heading_Total_Observed_Current,...
                                                                                 Rudder_Angle_Commanded_Current,...
                                                                                 Wave_Pulsation_Estimated,...
                                                                                 Damping_Wave_Estimated,...
                                                                                 Time_Current,...
                                                                                 Time_Constant,...
                                                                                 Static_Gain,...
                                                                                 Time_Sampling,...
                                                                                 Noise_For_Heading_wave,...
                                                                                 Torque_Wind_Estimated_Input,...
                                                                                 Inertia_Ship_Vertical,...
                                                                                 Wave_Pulsation_Identified,...
                                                                                 Heading_Rate_Estimated_Current_Navigation,...
                                                                                 Damping_Wave_Identified);
else % Exponential matrix discretization:
    [Heading_Rate_Wave_Estimated_Current,...
     Heading_Wave_Estimated_Current,...
     Heading_Low_Frequency_Estimated_Current,...
     Heading_Rate_Estimated_Current,...
     Bias_Estimated_Current,...
     Covariance_Aposteriori_Estimate] = Kalman_Observer_Wave_Estimation_Discretization(Heading_Total_Observed_Current,...
                                                                                       Rudder_Angle_Commanded_Current,...
                                                                                       Wave_Pulsation_Estimated,...
                                                                                       Damping_Wave_Estimated,...
                                                                                       Time_Current,...
                                                                                       Time_Constant,...
                                                                                       Static_Gain,...
                                                                                       Time_Sampling,...
                                                                                       Noise_For_Heading_wave,...
                                                                                       Torque_Wind_Estimated_Input,...
                                                                                       Inertia_Ship_Vertical,...
                                                                                       Wave_Pulsation_Identified,...
                                                                                       Heading_Rate_Estimated_Current_Navigation);


end

== matlab function Simulator_Case_9/Navigation_Estimation_Filtering/Wave_Estimation_Perturbation/Wave_Identification_Parameters_ARMA ==
  data: Heading_Wave_High_Frequency_Estimated input; Wave_Pulsation_Estimated output; Wave_Damping_Factor_Estimated output; Time_Sampling input
function [Wave_Pulsation_Estimated,...
          Wave_Damping_Factor_Estimated] = Wave_Parameters_Identification_ARMA(Heading_Wave_High_Frequency_Estimated,...
                                                                               Time_Sampling)

% Two stage Recursive Extended least squares algorithm to estimate the wave
% pulsation and damping factor:
[Wave_Pulsation_Estimated,...
 Wave_Damping_Factor_Estimated] = Wave_Identification_ARMA(Heading_Wave_High_Frequency_Estimated,...
                                                           Time_Sampling);


end

== matlab function Simulator_Case_9/Navigation_Estimation_Filtering/Wave_Estimation_Perturbation/High_Pass_Filter ==
  data: Heading_Unfiltered_Input input; Heading_Filtered_Ouput output; Time_Sampling input
function Heading_Filtered_Ouput= High_Pass_Wave_Filter(Heading_Unfiltered_Input,...
                                                       Time_Sampling)

% Online numerical high-pass filter for pre-processing of the heading for
% identification:
Heading_Filtered_Ouput = High_Pass_Wave_Filter_Identification(Heading_Unfiltered_Input,...
                                                              Time_Sampling);

end

== matlab function Simulator_Case_9/Controller_Actuator/Controller/PDF_Controller ==
  data: Heading_Aimed_Current input; Rudder_Angle_Elaborated_Current output; Heading_Observed_Current input; Velocity_Current input; Gain_Filter input; Damping_Aimed input; Pulsation_Aimed input; Time_Sampling input; Length_Ship_Current input; Density_Water_Current input; Drag_Coefficient_Current input; Draft_Depth_Current input; Longeron_Area_Current input; Mass_Of_The_Ship_Current input; Velocity_Initial input
function Rudder_Angle_Elaborated_Current = PDF_Controller(Heading_Aimed_Current,...
                                                          Heading_Observed_Current,...
                                                          Velocity_Current,...
                                                          Gain_Filter,...
                                                          Damping_Aimed,...
                                                          Pulsation_Aimed,...
                                                          Time_Sampling,...
                                                          Length_Ship_Current,...
                                                          Density_Water_Current,...
                                                          Drag_Coefficient_Current,...
                                                          Draft_Depth_Current,...
                                                          Longeron_Area_Current,...
                                                          Mass_Of_The_Ship_Current,...
                                                          Velocity_Initial)

% Adaptative controller:
Rudder_Angle_Elaborated_Current = Controller_PDF_LPV_Velocity(Heading_Aimed_Current,...
                                                              Heading_Observed_Current,...
                                                              Velocity_Current,...
                                                              Gain_Filter,...
                                                              Damping_Aimed,...
                                                              Pulsation_Aimed,...
                                                              Time_Sampling,...
                                                              Length_Ship_Current,...
                                                              Density_Water_Current,...
                                                              Drag_Coefficient_Current,...
                                                              Draft_Depth_Current,...
                                                              Longeron_Area_Current,...
                                                              Mass_Of_The_Ship_Current,...
                                                              Velocity_Initial);

end

== matlab function Simulator_Case_9/Navigation_Estimation_Filtering/Heading_Sensor_Fusion ==
  settings: updateMethod=DISCRETE
  data: Position_Ship_X_Current_GPS input; Position_Ship_Y_Current_GPS input; Heading_GPS input; Heading_Magnetometer input; Position_Ship_X_Current_Filtered output; Position_Ship_Y_Current_Filtered output; Heading_Ship_Current_Filtered output; Heading_Rate_Current_Filtered output; Velocity_Ship_GPS input; Time_Sampling input; Rudder_Angle_Elaborated input; Bias_Heading_Rate_Current_Model output; Velocity_Ship_Current output; Length_Ship_Current input; Density_Water_Current input; Drag_Coefficient_Current input; Draft_Depth_Current input; Longeron_Area_Current input; Mass_Of_The_Ship_Current input; Velocity_Ship_Initial input; Position_X_Ship_Initial input; Position_Y_Ship_Initial input
function [Position_Ship_X_Current_Filtered,...
          Position_Ship_Y_Current_Filtered,...
          Heading_Ship_Current_Filtered,...
          Heading_Rate_Current_Filtered,...
          Bias_Heading_Rate_Current_Model,...
          Velocity_Ship_Current] = Navigation_Kalman_Sensor_Fusion(Position_Ship_X_Current_GPS,...
                                                                   Position_Ship_Y_Current_GPS,...
                                                                   Heading_GPS,...
                                                                   Heading_Magnetometer,...
                                                                   Velocity_Ship_GPS,...
                                                                   Time_Sampling,...
                                                                   Rudder_Angle_Elaborated,...
                                                                   Length_Ship_Current,...
                                                                   Density_Water_Current,...
                                                                   Drag_Coefficient_Current,...
                                                                   Draft_Depth_Current,...
                                                                   Longeron_Area_Current,...
                                                                   Mass_Of_The_Ship_Current,...
                                                                   Velocity_Ship_Initial,...
                                                                   Position_X_Ship_Initial,...
                                                                   Position_Y_Ship_Initial)

% This function serves as a filtering and data fusion to provide the ship
% with the right heading data.
[Position_Ship_X_Current_Filtered,...
 Position_Ship_Y_Current_Filtered,...
 Heading_Ship_Current_Filtered,...
 Heading_Rate_Current_Filtered,...
 Bias_Heading_Rate_Current_Model,...
 Velocity_Ship_Current] = EKF_Heading_Position_Velocity(Position_Ship_X_Current_GPS,...
                                                        Position_Ship_Y_Current_GPS,...
                                                        Heading_GPS,...
                                                        Heading_Magnetometer,...
                                                        Velocity_Ship_GPS,...
                                                        Time_Sampling,...
                                                        Rudder_Angle_Elaborated,...
                                                        Length_Ship_Current,...
                                                        Density_Water_Current,...
                                                        Drag_Coefficient_Current,...
                                                        Draft_Depth_Current,...
                                                        Longeron_Area_Current,...
                                                        Mass_Of_The_Ship_Current,...
                                                        Velocity_Ship_Initial,...
                                                        Position_X_Ship_Initial,...
                                                        Position_Y_Ship_Initial);


end
